simulink model "d1_vanderpol"  (R2013a)
settings: Solver=ode45  StartTime=0.0  StopTime=80  RelTol=1e-3
settings Model: Creator=Lazaros  LastModifiedBy=Lazaros
settings DataIOCC: LimitDataPoints=off  Refine=4

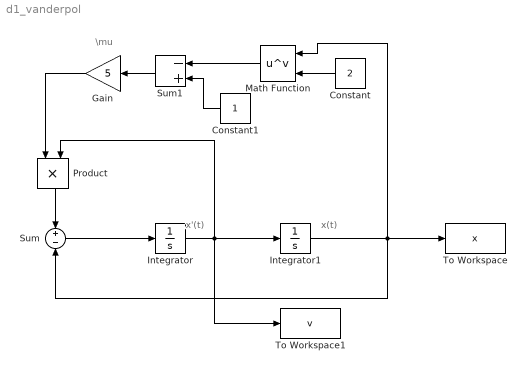
== system d1_vanderpol ==
  note: \mu
  note: x'(t)
  note: x(t)
  Constant : Constant  Value=2
  Constant1 : Constant
  Gain : Gain  Gain=5
  Integrator : Integrator  InitialCondition=1
  Integrator1 : Integrator  InitialCondition=2
  Math Function : Math  Operator=pow  SaturateOnIntegerOverflow=on
  Product : Product
  Sum : Sum  Inputs=+-
  Sum1 : Sum  Inputs=-+
  To Workspace : ToWorkspace  VariableName=x  SampleTime=-1
  To Workspace1 : ToWorkspace  VariableName=v  SampleTime=-1
  wires:
  Sum/1 -> Integrator/1
  Integrator/1 -> Product/2, To Workspace1/1, Integrator1/1
  Integrator1/1 -> Math Function/1, To Workspace/1, Sum/2
  Math Function/1 -> Sum1/1
  Constant1/1 -> Sum1/2
  Sum1/1 -> Gain/1
  Gain/1 -> Product/1
  Product/1 -> Sum/1
  Constant/1 -> Math Function/2
